simulink model "Controllo_beta3"  (Simulink 7.8)
settings: Solver=ode45  StartTime=0.0  StopTime=100  RelTol=1e-7
settings Model: Creator=dAnIeLe  LastModifiedBy=dAnIeLe
settings DebuggingCC: SolverPrmCheckMsg=none

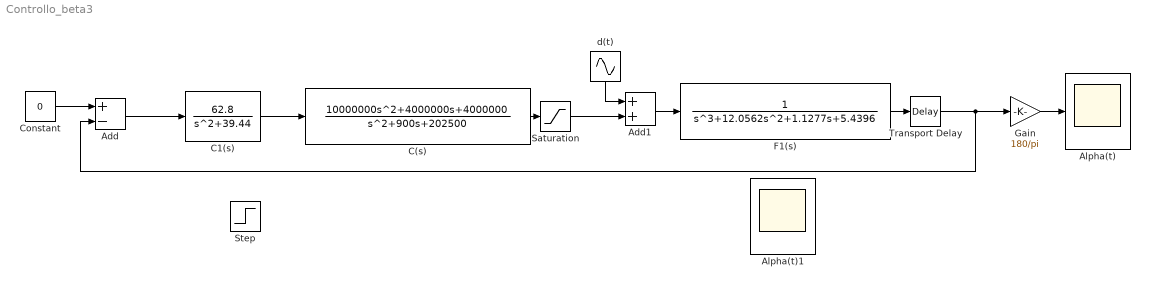
== system Controllo_beta3 ==
  Add : Sum  Inputs=+-
  Add1 : Sum
  Alpha(t) : Scope
      settings: TimeRange=15  YMin=-7e+89  YMax=6e+89
  Alpha(t)1 : Scope
      settings: TimeRange=15  YMin=-7e+89  YMax=6e+89
  C(s) : TransferFcn  Numerator=[10000000 4000000 4000000]  Denominator=[1 900 202500]
  C1(s) : TransferFcn  Numerator=[62.8]  Denominator=[1 0 39.44]
  Constant : Constant  Value=0
  F1(s) : TransferFcn  Denominator=[1 12.0562 1.1277 5.4396]
  Gain : Gain  Gain=180/pi
  Saturation : Saturate  UpperLimit=0.038  LowerLimit=0.033
  Step : Step  SampleTime=0
  Transport Delay : TransportDelay  DelayTime=0.00002  BufferSize=4096
  d(t) : Sin  Amplitude=0.1  Frequency=0.628  SampleTime=0
  wires:
  Constant/1 -> Add/1
  Transport Delay/1 -> Add/2, Gain/1
  Gain/1 -> Alpha(t)/1
  F1(s)/1 -> Transport Delay/1
  d(t)/1 -> Add1/1
  Add1/1 -> F1(s)/1
  C1(s)/1 -> C(s)/1
  Saturation/1 -> Add1/2
  C(s)/1 -> Saturation/1
  Add/1 -> C1(s)/1
